simulink model "GlbDa_SetData"  (R2016b)
settings: configuration reference "CodeGenConfigSet" (kept outside this file)
values from neighbouring files (symbols this model uses):
  TrbCh_n_C = Calibration.Parameter    [init_GlbDa_SetData.m]
settings Model: Creator=Wollf  LastModifiedBy=lenovo
settings ConfigSetRef: SourceLocation=Base Workspace

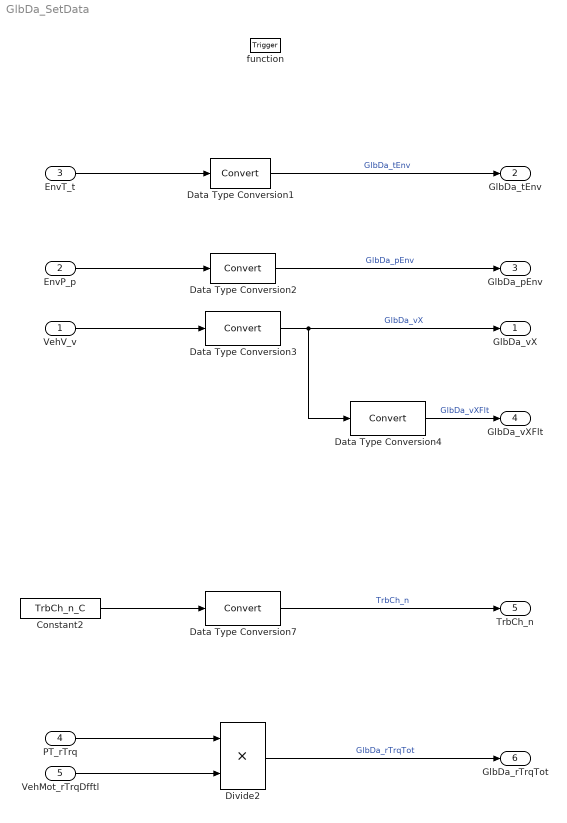
== system GlbDa_SetData ==
  VehV_v : Inport  Tag=km/h  Description=Vehicle speed  OutMin=0  OutMax=250  OutDataTypeStr=VehSpeed_km_h
  EnvP_p : Inport  Tag=kPa  Description=Barometric pressure  Port=2  OutMin=0  OutMax=3276  OutDataTypeStr=AirPressure_kPa
  EnvT_t : Inport  Tag=deg  Description=Environmental temperature  Port=3  OutMin=-200  OutMax=200  OutDataTypeStr=Temp_deg
  PT_rTrq : Inport  Description=Powertrain torque ratio  Port=4  OutMin=-100  OutMax=100  OutDataTypeStr=TransRatio
  VehMot_rTrqDfftl : Inport  Description=Torque ratio of differential  Port=5  OutMin=-300  OutMax=300  OutDataTypeStr=TransRatio
  function : TriggerPort  TriggerType=function-call  VariantControl=Variant
  Constant2 : Constant  Value=TrbCh_n_C
  Data Type Conversion{1..4,7} (5 alike) : DataTypeConversion
  Divide2 : Product  Inputs=**  OutDataTypeStr=Inherit: Inherit via back propagation  SaturateOnIntegerOverflow=on
  GlbDa_vX : Outport  Tag=km/h  Description=Longitudinal vehicle speed (X-direction)  OutMin=0  OutMax=250  OutDataTypeStr=VehSpeed_km_h
  GlbDa_tEnv : Outport  Tag=deg  Description=environment temperature  Port=2  OutMin=-50  OutMax=150  OutDataTypeStr=Temp_deg
  GlbDa_pEnv : Outport  Tag=kPa  Description=environmental pressure  Port=3  OutMin=-3000  OutMax=3000  OutDataTypeStr=AirPressure_kPa
  GlbDa_vXFlt : Outport  Tag=km/h  Description=Vehicle velocity filtered  Port=4  OutMin=0  OutMax=250  OutDataTypeStr=VehSpeed_km_h
  TrbCh_n : Outport  Tag=rpm  Description=Turbo charger speed  Port=5  OutMin=-327679  OutMax=327671  OutDataTypeStr=Turbo_rpm
  GlbDa_rTrqTot : Outport  Description=total ratio of the power train inclusive the differential and the converter torque ratio  Port=6  OutMin=-327  OutMax=327  OutDataTypeStr=TransRatio
  wires:
  Data Type Conversion1/1 -> GlbDa_tEnv/1  "GlbDa_tEnv"
  Data Type Conversion2/1 -> GlbDa_pEnv/1  "GlbDa_pEnv"
  Data Type Conversion3/1 -> GlbDa_vX/1, Data Type Conversion4/1  "GlbDa_vX"
  VehV_v/1 -> Data Type Conversion3/1
  Data Type Conversion4/1 -> GlbDa_vXFlt/1  "GlbDa_vXFlt"
  Constant2/1 -> Data Type Conversion7/1
  Data Type Conversion7/1 -> TrbCh_n/1  "TrbCh_n"
  VehMot_rTrqDfftl/1 -> Divide2/2
  Divide2/1 -> GlbDa_rTrqTot/1  "GlbDa_rTrqTot"
  PT_rTrq/1 -> Divide2/1
  EnvT_t/1 -> Data Type Conversion1/1
  EnvP_p/1 -> Data Type Conversion2/1
